simulink model "classActivity"  (R2023b)
settings: Solver=FixedStepAuto  StartTime=0.0  StopTime=10.0  FixedStep=0.01  RelTol=1e-3
settings Model: Creator=qasem  LastModifiedBy=Fartash
settings OptimizationCC: DefaultParameterBehavior=Inlined  EnhancedBackFolding=on  PassReuseOutputArgsAs=Individual arguments  ZeroExternalMemoryAtStartup=off  ZeroInternalMemoryAtStartup=off  MaxStackSize=64  OptimizeBlockOrder=speed  DifferentSizesBufferReuse=on  OptimizationCustomize=off  EfficientTunableParamExpr=on
settings DebuggingCC: ParameterTunabilityLossMsg=error
settings HardwareCC: ProdBitPerInt=16  ProdBitPerPointer=16  ProdBitPerSizeT=16  ProdBitPerPtrDiffT=16  ProdLargestAtomicFloat=None  ProdWordSize=8  ProdHWDeviceType=Atmel->AVR
settings SFSimCC: MATLABDynamicMemAlloc=off
settings RTWCC: Description=Embedded Coder  SystemTargetFile=ert.tlc  GenCodeOnly=on  TemplateMakefile=ert_default_tmf  Toolchain=MinGW64 | gmake (64-bit Windows)  BuildConfiguration=Faster Runs  TargetLang=C++
settings CodeAppCC: ForceParamTrailComments=on  IgnoreCustomStorageClasses=off  OperatorAnnotations=on  SimulinkDataObjDesc=on  SFDataObjDesc=on  InsertBlockDesc=on
settings ERTTargetCC: TargetLangStandard=C++11 (ISO)  CodeInterfacePackaging=C++ class  SupportContinuousTime=on  ExtModeTransport=3  ExtModeStaticAlloc=on  ExtModeStaticAllocSize=250  ExtModeMexFile=ext_xcp  ExtModeIntrfLevel=Level2 - Open  RootIOFormat=Structure reference  ERTCustomFileTemplate=example_file_process.tlc
settings ConfigComp: CovEnable=on  RecordCoverage=on  CovModelRefEnable=on

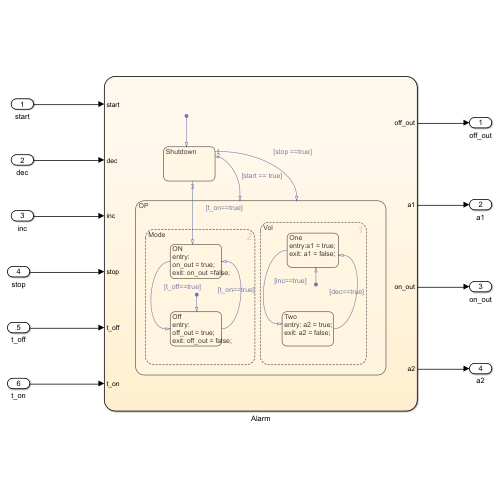
[thumbnail: Simulink's stored preview of the top-level diagram]
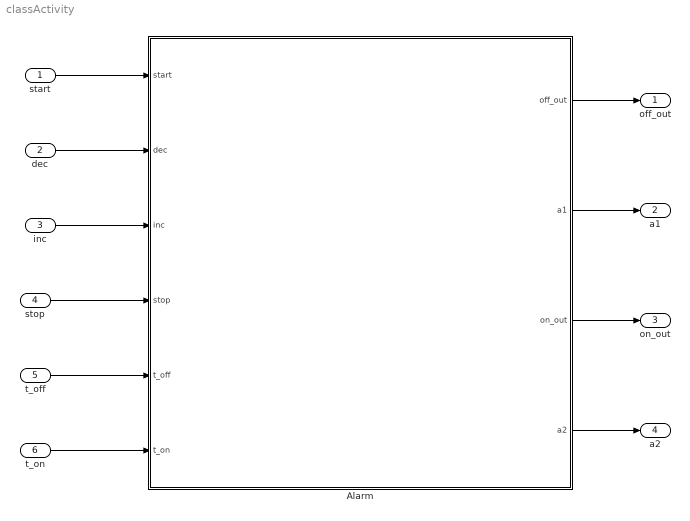
== system classActivity ==
  start : Inport
  dec : Inport  Port=2
  inc : Inport  Port=3
  stop : Inport  Port=4
  t_off : Inport  Port=5
  t_on : Inport  Port=6
  Alarm : Stateflow chart  TreatAsAtomicUnit=on
      settings: PortSchema="{\"entries\":[{\"content\":{\"sides\":[{\"content\":{\"connectorIds\":[\"In1\",\"In2\",\"In3\",\"In4\",\"In5\",\"In6\"]},\"type\":\"ConnectorPlacement.EquallySpacedRectSide\",\"uuid\":\"67fa7592-dd5f-473b-adb5-31a8a36dc656\"},{\"content\":{\"connectorIds\":[\"Out1\",\"Out3\",\"Out2\",\"Out4\"],\"side\":\"RIGHT\"},\"type\":\"ConnectorPlacement.EquallySpacedRectSide\",\"uuid\":\"ab42aef1-4252-4a8b-8856-fd08774fb9b6\"},{\"content\":{\"side\":\"TOP\"},\"type\":\"ConnectorPlacement.EquallySpacedRectSide\",\"uuid\":\"0f3ec35b-95fb-46bd-8956-4d67cc055612\"}]},\"type\":\"ConnectorPlacement.EquallySpacedConnector\",\"uuid\":\"eed7d48e-0090-434b-a77a-4ae4108e4a5f\"}],\"packageUris\":[\"http://schema.mathworks.com/mf0/Connector/R2020b\"],\"version\":\"1.0\"}"
  off_out : Outport
  a1 : Outport  Port=2
  on_out : Outport  Port=3
  a2 : Outport  Port=4
  wires:
  Alarm/1(off_out) -> off_out/1
  Alarm/3(a1) -> a1/1
  Alarm/2(on_out) -> on_out/1
  Alarm/4(a2) -> a2/1
  start/1 -> Alarm/1(start)
  dec/1 -> Alarm/2(dec)
  inc/1 -> Alarm/3(inc)
  stop/1 -> Alarm/4(stop)
  t_off/1 -> Alarm/5(t_off)
  t_on/1 -> Alarm/6(t_on)

== stateflow chart classActivity/Alarm ==
  state Shutdown
  state OP
    state Vol [parallel]
      settings: executionOrder=2
      state One
        entry:a1 = true;
        a2 = false;
      state Two
        entry: a2 = true;
        a1 = false;
      One -> Two : [inc==true && dec==false && start == true]
      Two -> One : [dec==true && inc == false && start == true]
      (default) -> One
    state Mode [parallel]
      settings: executionOrder=1
      state ON
        entry:
        on_out = true;
        off_out =false;
      state Off
        entry:
        off_out = true;
        on_out = false;
      Off -> ON : [t_on==true && t_off == false]
      ON -> Off : [t_off==true && t_on==false]
      (default) -> Off
  (default) -> Shutdown : {a1= false; a2= false; on_out=false; off_out=false;}
  Shutdown -> OP [order 1] : [start == true && stop == false]
  OP -> Shutdown : [stop ==true || start == false]{a1= false; a2= false; on_out=false; off_out=false;}
  Shutdown -> ON [order 2] : [t_on==true && stop == false]{ a1= false; a2=false}
  data: start input boolean; dec input boolean; inc input boolean; stop input boolean; t_off input boolean; t_on input boolean; off_out output boolean; on_out output boolean; a1 output boolean; a2 output boolean
